simulink model "TLNWithUnrealTestBench"  (R2023a)
settings: Solver=FixedStepAuto  StartTime=0.0  StopTime=15  FixedStep=0.001  RelTol=1e-8  EnableMultiTasking=on
PostLoadFcn:
  | helperSLTrafficLightNegotiationWithUnrealSetup
values from neighbouring files (symbols this model uses):
  vehSim3D = repmat(     struct(     'Length', 0,     'InitialPos',[0 0 0],     'InitialRot',[0 0 0]),     numVehicles,1)    [helperSLTrafficLightNegotiationWithUnrealSetup.m]
undefined symbols (not defined in the file or in its folder): Curvature, CurvatureDerivative, driving, gray, HeadingAngle, intersectionInfo, LateralOffset, Left, M, matlabshared, N, referencePathInfo, Right, setVelocity, Strength, trafficLightConfig, Ts
libraries: drivingscenarioandsensors x8, sim3dautolib x4, visionanalysis x2, sim3dcameralib x2, sim3dlib x1, helperTrafficLightControllerLib x1, dspvision x1, trackingutilitieslib x1, drivinglib x1
CloseFcn:
  | helperSLTrafficLightNegotiationWithUnrealCleanUp
settings Model: Creator=The MathWorks, Inc.  LastModifiedBy=david
settings SolverCC: ZeroCrossAlgorithm=Adaptive  AlgebraicLoopSolver=TrustRegion  PositivePriorityOrder=on  AutoInsertRateTranBlk=on  InsertRTBMode=Always  DecoupledContinuousIntegration=on  MinimalZcImpactIntegration=on  MaxZcPerStep=1
settings DataIOCC: SaveOutput=off  SaveTime=off  ReturnWorkspaceOutputs=off
settings OptimizationCC: DefaultParameterBehavior=Inlined  EnhancedBackFolding=on  PassReuseOutputArgsAs=Individual arguments  ZeroExternalMemoryAtStartup=off  ZeroInternalMemoryAtStartup=off  OptimizeBlockOrder=speed  DifferentSizesBufferReuse=on  OptimizationCustomize=off  EfficientTunableParamExpr=on
settings DebuggingCC: MaskedZcDiagnostic=none  IgnoredZcDiagnostic=none  ParameterPrecisionLossMsg=none  ParameterTunabilityLossMsg=error  UnconnectedInputMsg=warning  UnconnectedOutputMsg=warning  UnconnectedLineMsg=warning  PregeneratedLibrarySubsystemCodeDiagnostic=none  ArithmeticOperatorsInVariantConditions=warning
settings HardwareCC: ProdLongLongMode=on
settings ModelReferenceCC: EnableRefExpFcnMdlSchedulingChecks=on
settings SFSimCC: SimUseLocalCustomCode=off
settings RTWCC: Description=Embedded Coder  SystemTargetFile=ert.tlc  TemplateMakefile=ert_default_tmf  GenerateReport=on  RTWUseLocalCustomCode=off  LaunchReport=on  DLArmComputeVersion=19.05
settings CodeAppCC: ForceParamTrailComments=on  IgnoreCustomStorageClasses=off  OperatorAnnotations=on  SimulinkDataObjDesc=on  SFDataObjDesc=on  InsertBlockDesc=on
settings ERTTargetCC: TargetLangStandard=C99 (ISO)  GenerateSampleERTMain=on  InlinedParameterPlacement=NonHierarchical  ERTCustomFileTemplate=example_file_process.tlc
settings ConfigComp: CovScope=ReferencedModels  CovIncludeTopModel=off

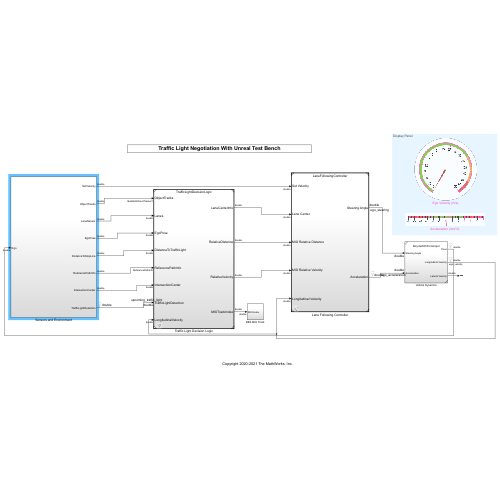
[thumbnail: Simulink's stored preview of the top-level diagram]
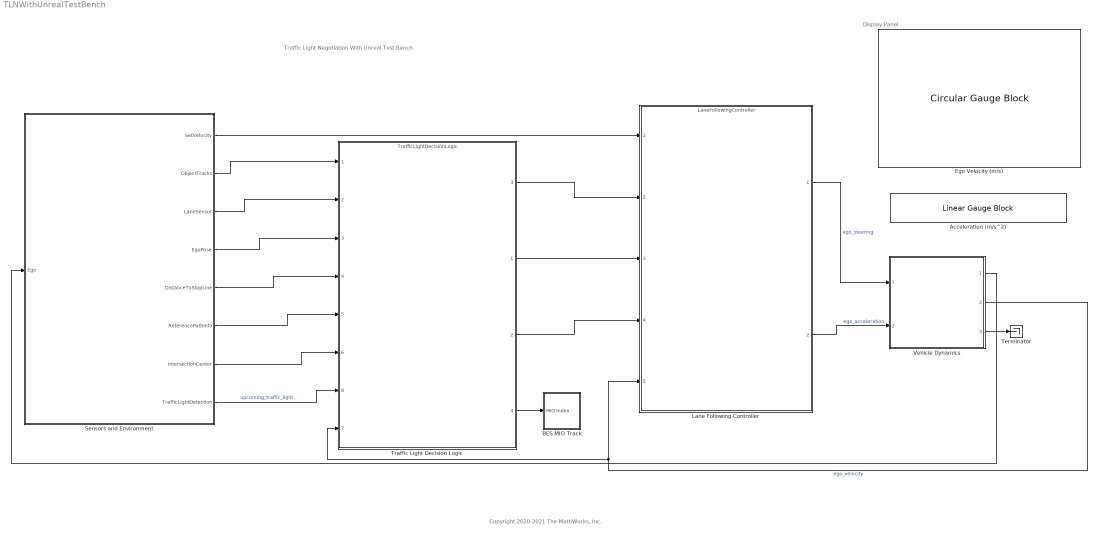
== system TLNWithUnrealTestBench ==
  note: Traffic Light Negotiation With Unreal Test Bench
  note: Display Panel
  note: Copyright 2020-2021 The MathWorks, Inc.
  Acceleration (m/s^2) : LinearGaugeBlock  LabelPosition=Hide  ScaleMin=-6  ScaleMax=6
  BES MIO Track : Subsystem
  Ego Velocity (m/s) : CircularGaugeBlock  LabelPosition=Hide  ScaleMax=50
  Lane Following Controller : ModelReference  ModelNameDialog=LaneFollowingController.slx  SimulationMode=Normal  ModelReferenceVersion=7.0
  Sensors and Environment : Subsystem
  Terminator : Terminator
  Traffic Light Decision Logic : ModelReference  ModelNameDialog=TrafficLightDecisionLogic  SimulationMode=Normal  ModelReferenceVersion=6.4
      settings: PortSchema="{\"entries\":[{\"content\":{\"sides\":[{\"content\":{\"connectorIds\":[\"In1\",\"In2\",\"In3\",\"In4\",\"In5\",\"In6\",\"In8\",\"In7\"]},\"type\":\"ConnectorPlacement.EquallySpacedRectSide\",\"uuid\":\"80441088-7f88-498e-bd57-56a9591db5ab\"},{\"content\":{\"connectorIds\":[\"Out3\",\"Out1\",\"Out2\",\"Out4\"],\"side\":\"RIGHT\"},\"type\":\"ConnectorPlacement.EquallySpacedRectSide\",\"uuid\":\"71bac071-b53b-4fb3-8fe7-17db6e81a6fe\"},{\"content\":{\"side\":\"TOP\"},\"type\":\"ConnectorPlacement.EquallySpacedRectSide\",\"uuid\":\"95fcddf4-1608-4cb5-a6ec-8633d9712dcc\"},{\"content\":{\"side\":\"HIDDEN\"},\"type\":\"ConnectorPlacement.EquallySpacedRectSide\",\"uuid\":\"8d5e9fdd-dbcd-4e58-97a7-7da238f3d39d\"}]},\"type\":\"ConnectorPlacement.EquallySpacedConnector\",\"uuid\":\"78ce1c2f-8a23-470e-877e-968badbfaf17\"}],\"packageUris\":[\"http://schema.mathworks.com/mf0/Connector/R2020b\"],\"version\":\"1.0\"}"
  Vehicle Dynamics : Subsystem  ReferencedSubsystem=BicycleWithForceInput
  wires:
  Sensors and Environment/2(ObjectTracks) -> Traffic Light Decision Logic/1
  Sensors and Environment/1(SetVelocity) -> Lane Following Controller/1
  Sensors and Environment/8(TrafficLightDetection) -> Traffic Light Decision Logic/8  "upcoming_traffic_light"
  Vehicle Dynamics/1 -> Sensors and Environment/1(Ego)
  Sensors and Environment/4(EgoPose) -> Traffic Light Decision Logic/3
  Sensors and Environment/3(LaneSensor) -> Traffic Light Decision Logic/2
  Sensors and Environment/5(DistanceToStopLine) -> Traffic Light Decision Logic/4
  Sensors and Environment/6(ReferencePathInfo) -> Traffic Light Decision Logic/5
  Sensors and Environment/7(IntersectionCenter) -> Traffic Light Decision Logic/6
  Lane Following Controller/1 -> Vehicle Dynamics/1  "ego_steering"
  Lane Following Controller/2 -> Vehicle Dynamics/2  "ego_acceleration"
  Traffic Light Decision Logic/3 -> Lane Following Controller/2
  Traffic Light Decision Logic/1 -> Lane Following Controller/3
  Traffic Light Decision Logic/2 -> Lane Following Controller/4
  Traffic Light Decision Logic/4 -> BES MIO Track/1(MIO Index)
  Vehicle Dynamics/2 -> Lane Following Controller/5, Traffic Light Decision Logic/7  "ego_velocity"
  Vehicle Dynamics/3 -> Terminator/1

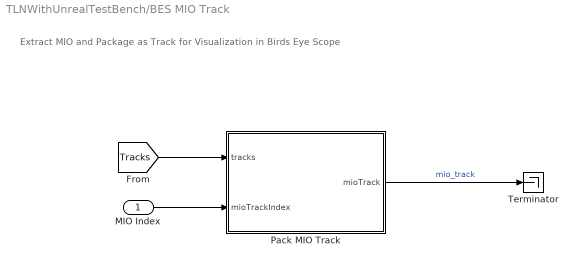
== system TLNWithUnrealTestBench/BES MIO Track ==
  note: Extract MIO and Package as Track for Visualization in Birds Eye Scope
  MIO Index : Inport
  Pack MIO Track : MATLAB Function  TreatAsAtomicUnit=on
  Terminator : Terminator
  wires:
  MIO Index/1 -> Pack MIO Track/2(mioTrackIndex)
  [Tracks] -> Pack MIO Track/1(tracks)
  Pack MIO Track/1(mioTrack) -> Terminator/1  "mio_track"

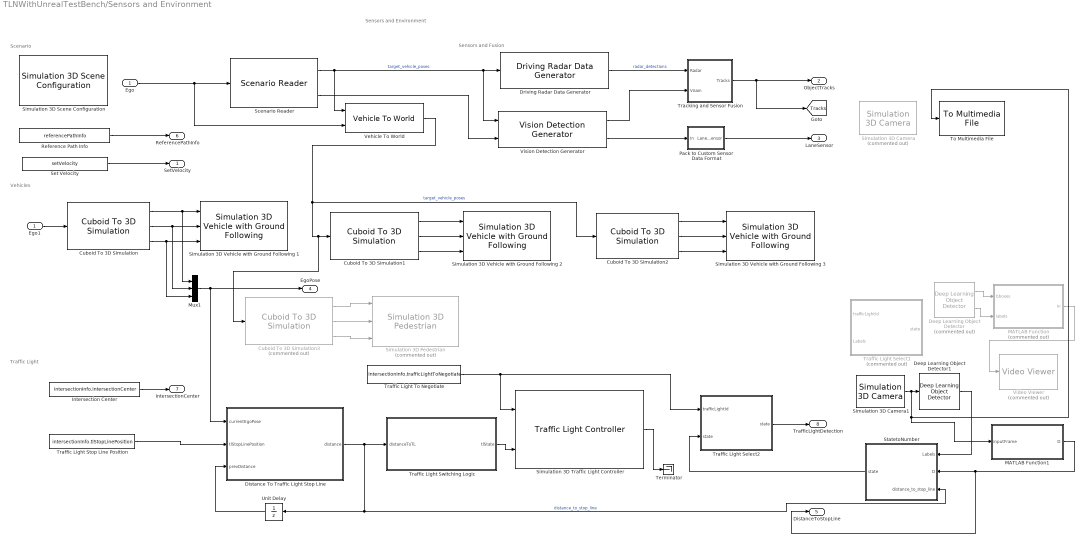
== system TLNWithUnrealTestBench/Sensors and Environment ==
  note: Sensors and Fusion
  note: Traffic Light
  note: Scenario
  note: Sensors and Environment
  note: Vehicles
  Ego : Inport
  Cuboid To 3D Simulation : drivingscenarioandsensors/Cuboid To 3D Simulation  SpecifyActorID=off  ActorIDToConvert=1  SimulateUsing=Interpreted execution
  Cuboid To 3D Simulation1 : drivingscenarioandsensors/Cuboid To 3D Simulation  SpecifyActorID=on  ActorIDToConvert=68  SimulateUsing=Interpreted execution
  Cuboid To 3D Simulation2 : drivingscenarioandsensors/Cuboid To 3D Simulation  SpecifyActorID=on  ActorIDToConvert=69  SimulateUsing=Interpreted execution
  Cuboid To 3D Simulation3 : drivingscenarioandsensors/Cuboid To 3D Simulation  Commented=on  SpecifyActorID=on  ActorIDToConvert=70  SimulateUsing=Interpreted execution
  Deep Learning Object Detector : visionanalysis/Deep Learning Object Detector  Commented=on  Detector=Detector from MAT-file  DetectorFunction=untitled  DetectorFilePath=C:\Users\david\Documents\MATLAB\TLNUnreal\TLNUnreal\TestAnalysis\Training_GYR\DetectorYolov2.mat  MaxDetections=500  Bboxes=on  Scores=off  UseROI=off  ROI=[1 1 100 100]  Threshold=0.5  NumStrongestRegions=2000  UseMinSize=off  MinSize=[1 1]  UseMaxSize=off  MaxSize=[50 50]  ForceInterpretedSim=off
  Deep Learning Object Detector1 : visionanalysis/Deep Learning Object Detector  Detector=Detector from MAT-file  DetectorFunction=untitled  DetectorFilePath=C:\Users\david\Documents\MATLAB\TLNUnreal\TLNUnreal\NoState\detectorYolo2.mat  MaxDetections=500  Bboxes=off  Scores=off  UseROI=off  ROI=[1 1 100 100]  Threshold=0.5  NumStrongestRegions=2000  UseMinSize=off  MinSize=[1 1]  UseMaxSize=off  MaxSize=[50 50]  ForceInterpretedSim=off
  Distance To Traffic Light Stop Line : MATLAB Function  TreatAsAtomicUnit=on  mask{minTLDist=3}
      mask prompts: minTLDist "Minimum distance to traffic light"
  Driving Radar Data Generator : drivingscenarioandsensors/Driving Radar Data Generator  SensorIndex=2  UpdateRate=10  MountingLocation=[ 0, 0.5, 0.2 ]  MountingAngles=[0 0 0]  HasElevation=off  HasRangeRate=on  HasNoise=off  HasFalseAlarms=off  HasOcclusion=on  MaxNumReportsSource=Property  MaxNumReports=50  TargetReportFormat=Clustered detections  DetectionCoordinates=Body  TrackCoordinates=Body  BusNameSource=Property  BusName=BusRadar  AzimuthResolution=4  ElevationResolution=5  RangeResolution=2.5  RangeRateResolution=0.5  AzimuthBiasFraction=0.1  ElevationBiasFraction=0.1  RangeBiasFraction=0.05  RangeRateBiasFraction=0.05  FieldOfView=[40, 5 ]  RangeLimits=[ 0, 174 ]  RangeRateLimits=[ -100, 100 ]  DetectionProbability=0.9  FalseAlarmRate=1e-06  ReferenceRange=100  ReferenceRCS=0  CenterFrequency=77e9  FilterInitializationFcn=initcvekf  ConfirmationThreshold=[2 3]  DeletionThreshold=[5 5]  InitialSeedSource=Repeatable  InitialSeed=0  UsedSeed=matlabshared.tracking.internal.SimulinkUtilities.seedManager(gcb)  ProfilesSource=From Scenario Reader block  ProfilesParameters=driving.internal.ActorProfilesRadarParameters  ProfilesExpression=struct('ClassID',0,'Length',4.7,'Width',1.8,'Height',1.4,'OriginOffset',[-1.35 0 0],'RCSPattern',[10 10;10 10],'RCSAzimuthAngles',[-180 180],'RCSElevationAngles',[-90 90])
  Ego1 : InportShadow
  Intersection Center : Constant  Value=intersectionInfo.intersectionCenter  SampleTime=Ts
  MATLAB Function : MATLAB Function  Commented=on  TreatAsAtomicUnit=on
  MATLAB Function1 : MATLAB Function  TreatAsAtomicUnit=on
  Mux1 : Mux  Inputs=3
  Pack to Custom Sensor Data Format : Subsystem
  Reference Path Info : Constant  Value=referencePathInfo  OutDataTypeStr=Bus: ReferencePathInfo  SampleTime=Ts
  Scenario Reader : drivingscenarioandsensors/Scenario Reader  ScenarioSource=From workspace  ScenarioFileName=C:\Users\david\Documents\MATLAB\TLNUnreal\TLNUnreal\TestScenarios\90DegreesStraight.mat  ScenarioVariableName=scenario_02_TLN_straight_greenToRed  OutputCoordinateSystem=Vehicle coordinates  EgoVehicleSource=Input port  EgoVehicleActorID=egoVehicle.ActorID  OrientVehiclesOnRoad=on  OutputEgoVehiclePose=off  OutputEgoVehicleState=off  SampleTime=Ts  LaneBoundaryOutput=All lane boundaries  LaneBoundaryDistance=0:0.5:60  LaneBoundaryLocation=Center of lane markings  BusNameSource=Auto  BusName=BusActors  BusNumActorsSource=Scenario  BusNumActors=100  BusName2Source=Auto  BusName2=BusLaneBoundaries  BusNumLaneBoundariesSource=Scenario  BusNumLaneBoundaries=10  BusName3Source=Auto  BusName3=BusEgoActor  BusName4Source=Auto  BusName4=BusEgoState  ShowCoordinateLabels=on  SimulateUsing=Interpreted execution
  Set Velocity : Constant  Value=setVelocity
  Simulation 3D Camera : sim3dcameralib/Simulation 3D Camera  Priority=1  Commented=on  sensorTag=Sim3dSensor3  sensorId=3  sensorName=Sim3dSensor3  vehTagList={'EgoVehicle';'Scene Origin';'SimulinkVehicle2';'SimulinkVehicle3'}  vehTag=EgoVehicle  mountLoc=Roof center  offsetFlag=off  tmountOffset=[0, 0, 0]  extTmount=off  rmountOffset=[0, 0, 0]  extRmount=off  FocalLength=[1109, 1109]  OpticalCenter=[640, 360]  ImageSize=[720, 1280]  RadialDistortion=[0, 0]  TangentialDistortion=[0, 0]  SensorSkew=0  DepthOutportEnabled=off  SemanticOutportEnabled=off  TransformOutportEnabled=off  SampleTime=-1  mountPoint=[-0.449999988079071 0 1.67999994754791]  mountOrientation=[0 0 0]  aMode=3  ID=3
      settings: LibrarySourceBlock=drivingsim3d/Simulation 3D Camera
  Simulation 3D Camera1 : sim3dcameralib/Simulation 3D Camera  Priority=1  sensorTag=Sim3dSensor2  sensorId=2  sensorName=Sim3dSensor2  vehTagList={'EgoVehicle';'Scene Origin';'SimulinkVehicle2';'SimulinkVehicle3'}  vehTag=EgoVehicle  mountLoc=Roof center  offsetFlag=off  tmountOffset=[0, 0, 0]  extTmount=off  rmountOffset=[0, 0, 0]  extRmount=off  FocalLength=[1109, 1109]  OpticalCenter=[640, 360]  ImageSize=[720, 1280]  RadialDistortion=[0, 0]  TangentialDistortion=[0, 0]  SensorSkew=0  DepthOutportEnabled=off  SemanticOutportEnabled=off  TransformOutportEnabled=off  SampleTime=-1  mountPoint=[-0.449999988079071 0 1.67999994754791]  mountOrientation=[0 0 0]  aMode=3  ID=2
      settings: LibrarySourceBlock=drivingsim3d/Simulation 3D Camera
  Simulation 3D Pedestrian : sim3dautolib/Simulation 3D Pedestrian  Priority=-1  Commented=on  PedestrianType=Male 1  Scale=[1, 1, 1]  InitialPos=[-55.1, -4, 0]  InitialYaw=0  ActorName=SimulinkPedestrian1  SampleTime=-1  ActorType=SimulinkPedestrian  ActorTag=SimulinkPedestrian1  ID=1  aMode=3  CoordinateScheme=ISO  TransformOutportEnabled=off
      settings: LibrarySourceBlock=drivingsim3d/Simulation 3D Pedestrian
  Simulation 3D Scene Configuration : sim3dlib/Simulation 3D Scene Configuration  Priority=0  ProjectFormat=Unreal Executable  SceneDesc=US city block  ProjectName=C:\Users\david\Documents\MATLAB\NoLightOn\WindowsNoEditor\AutoVrtlEnv.exe  ScenePath=/Game/Maps/USCityBlock  UEProjPath=C:\Users\david\Documents\MATLAB\AutoVrtlEnv - Copy\AutoVrtlEnv.uproject  EnableOpenDRIVE=off  vehTagList={'EgoVehicle';'Scene Origin';'SimulinkVehicle2';'SimulinkVehicle3'}  vehTag=EgoVehicle  OpVisEn=off  Ts=0.1  EnableWindow=on  EnableRemoteAccess=off  EnableWeather=off  SunAltitude=40.0  SunAzimuth=90  clouds=10  wind=1  fog=0  rain=0  EnableGeospatial=off  OriginHeight=200  OriginLatitude=40.744652  OriginLongitude=-73.988864  MapStyle=Aerial  AdditionalAssetIDs=[]  UseAdvancedSunSky=off  SolarTime=11  TimeZone=-5  Day=21  Month=9  Year=2022  UseDaylightSavingTime=on  DSTStartDay=10  DSTStartMonth=3  DSTEndDay=3  DSTEndMonth=11  DSTSwitchHour=2  sensorTag=MainCamera1  sensorId=1  sensorName=MainCamera1  mountLoc=Origin  offsetFlag=off  tmountOffset=[0, 0, 0]  rmountOffset=[0, 0, 0]  HorizontalResolution=1280  VerticalResolution=720  HorizontalFOV=60  mountPoint=[0 0 0]  mountOrientation=[0 0 0]  aMode=3  ID=1  GeoTrigger=Inactive
      settings: AttributesFormatString=SceneDesc = %<SceneDesc>
  Simulation 3D Traffic Light Controller : helperTrafficLightControllerLib/Traffic Light Controller  Priority=-1  helperTrafficLightCheck=0  customScene=0  modeType=State-based  vehTagList={'EgoVehicle';'Scene Origin';'SimulinkVehicle2';'SimulinkVehicle3'}  MsgSize=[1 62]  vehTag=EgoVehicle  trafficLightID=1  greenTime=10  yellowTime=3  redClearanceTime=0  aMode=3  Ts=-1
  Simulation 3D Vehicle with Ground Following 1 : sim3dautolib/Simulation 3D Vehicle with Ground Following  Priority=-1  PassVehMesh=Sedan  MeshPath=/MathWorksSimulation/Vehicles/Muscle/Meshes/SK_MuscleCar.SK_MuscleCar  TrackWidth=1.9  WheelBase=3  WheelRadius=0.35  VehColor=Blue  InitialPos=vehSim3D(1).InitialPos  InitialRot=vehSim3D(1).InitialRot  ActorName=EgoVehicle  SampleTime=-1  ActorType=SimulinkVehicle  ID=C  aMode=3  ActorTag=EgoVehicle  CoordinateScheme=ISO  VehLightsControl=off  HeadlightColor=[ 1, 1, 1 ]  HighBeamIntensity=100000  LowBeamIntensity=60000  HighBeamConeAngle=70  LowBeamConeAngle=70  LeftHeadlightOrientation=[ 0, 0 ]  RightHeadlightOrientation=[ 0, 0 ]  BrakelightIntensity=500  ReverselightIntensity=500  SignallightIntensity=500  SignallightPeriod=1  SignalPulseWidth=50  TransformOutportEnabled=off
      settings: AttributesFormatString=|
      | --------------------------------------
      | ActorName = %<ActorName>
      | PassVehMesh = %<PassVehMesh>
      | VehColor = %<VehColor>
  Simulation 3D Vehicle with Ground Following 2 : sim3dautolib/Simulation 3D Vehicle with Ground Following  Priority=-1  PassVehMesh=Sedan  MeshPath=/MathWorksSimulation/Vehicles/Muscle/Meshes/SK_MuscleCar.SK_MuscleCar  TrackWidth=1.9  WheelBase=3  WheelRadius=0.35  VehColor=Red  InitialPos=vehSim3D(2).InitialPos  InitialRot=vehSim3D(2).InitialRot  ActorName=SimulinkVehicle2  SampleTime=-1  ActorType=SimulinkVehicle  ID=2  aMode=3  ActorTag=SimulinkVehicle2  CoordinateScheme=ISO  VehLightsControl=off  HeadlightColor=[ 1, 1, 1 ]  HighBeamIntensity=100000  LowBeamIntensity=60000  HighBeamConeAngle=70  LowBeamConeAngle=70  LeftHeadlightOrientation=[ 0, 0 ]  RightHeadlightOrientation=[ 0, 0 ]  BrakelightIntensity=500  ReverselightIntensity=500  SignallightIntensity=500  SignallightPeriod=1  SignalPulseWidth=50  TransformOutportEnabled=off
      settings: AttributesFormatString=|
      | --------------------------------------
      | ActorName = %<ActorName>
      | PassVehMesh = %<PassVehMesh>
      | VehColor = %<VehColor>
  Simulation 3D Vehicle with Ground Following 3 : sim3dautolib/Simulation 3D Vehicle with Ground Following  Priority=-1  PassVehMesh=Muscle car  MeshPath=/MathWorksSimulation/Vehicles/Muscle/Meshes/SK_MuscleCar.SK_MuscleCar  TrackWidth=1.9  WheelBase=3  WheelRadius=0.35  VehColor=Black  InitialPos=vehSim3D(3).InitialPos  InitialRot=vehSim3D(3).InitialRot  ActorName=SimulinkVehicle3  SampleTime=-1  ActorType=SimulinkVehicle  ID=3  aMode=3  ActorTag=SimulinkVehicle3  CoordinateScheme=ISO  VehLightsControl=off  HeadlightColor=[ 1, 1, 1 ]  HighBeamIntensity=100000  LowBeamIntensity=60000  HighBeamConeAngle=70  LowBeamConeAngle=70  LeftHeadlightOrientation=[ 0, 0 ]  RightHeadlightOrientation=[ 0, 0 ]  BrakelightIntensity=500  ReverselightIntensity=500  SignallightIntensity=500  SignallightPeriod=1  SignalPulseWidth=50  TransformOutportEnabled=off
      settings: AttributesFormatString=|
      | --------------------------------------
      | ActorName = %<ActorName>
      | PassVehMesh = %<PassVehMesh>
      | VehColor = %<VehColor>
  StatetoNumber : MATLAB Function  TreatAsAtomicUnit=on
  Terminator : Terminator
  To Multimedia File : dspvision/To Multimedia File  outputFilename=C:\Users\david\Documents\MATLAB\Presentation\Gree,Yellow,Red.avi  streamSelection=Video only  videoCompressor=None (uncompressed)  audioCompressor=None (uncompressed)  imagePorts=One multidimensional signal  fileType=AVI  audioDatatype=Determine from input data type  fourcc=RGB  videoQuality=75  mj2000CompFactor=10
      settings: LibrarySourceBlock=visionsinks/To Multimedia File
  Tracking and Sensor Fusion : Subsystem  TreatAsAtomicUnit=on
      settings: RTWFileNameOpts=Use function name
  Traffic Light Select1 : MATLAB Function  Commented=on  TreatAsAtomicUnit=on
  Traffic Light Select2 : MATLAB Function  TreatAsAtomicUnit=on
  Traffic Light Stop Line Position : Constant  Value=intersectionInfo.tlStopLinePosition  OutDataTypeStr=double
  Traffic Light Switching Logic : Stateflow chart  TreatAsAtomicUnit=on  SystemSampleTime=Ts  mask{tlConfig=trafficLightConfig}
      mask prompts: tlConfig "Configuration Params"
  Traffic Light To Negotiate : Constant  Value=intersectionInfo.trafficLightToNegotiate
  Unit Delay : UnitDelay  InitialCondition=100  SampleTime=-1  HasFrameUpgradeWarning=on
  Vehicle To World : drivingscenarioandsensors/Vehicle To World  BusNameSource=Auto  BusName=BusVehicleToWorldActors  SimulateUsing=Interpreted execution
  Video Viewer : VideoViewer  Commented=on  colormapValue=gray(256)  FigPos=[1 726 1366 626]
  Vision Detection Generator : drivingscenarioandsensors/Vision Detection Generator  SensorIndex=1  DetectorOutput=Lanes and objects  UpdateInterval=0.1  LaneUpdateInterval=0.1  SensorLocation=[ 1.9, 0 ]  Height=1.1  Yaw=0  Pitch=1  Roll=0  BusNameSource=Property  BusName=BusVision  BusName2Source=Property  BusName2=BusLanes  MaxNumDetectionsSource=Property  MaxNumDetections=20  MaxNumLanesSource=Property  MaxNumLanes=2  DetectionCoordinates=Ego Cartesian  SimulateUsing=Interpreted execution  MaxRange=150  BoundingBoxAccuracy=5  ProcessNoiseIntensity=5  MaxSpeed=50  MaxAllowedOcclusion=0.5  MinObjectImageSize=[ 10, 10 ]  DetectionProbability=0.9  FalsePositivesPerImage=0.1  MinLaneImageSize=[ 20, 3 ]  LaneBoundaryAccuracy=3  HasNoise=on  InitialSeedSource=Repeatable  InitialSeed=0  UsedSeed=driving.internal.SimulinkUtilities.seedManager(gcb)  ActorProfilesSource=From Scenario Reader block  ActorProfilesParameters=driving.internal.ActorProfilesParameters  ActorProfilesExpression=struct( 'ClassID', 0, 'Length', 4.7, 'Width', 1.8, 'Height', 1.4, 'OriginOffset', [ -1.35, 0, 0 ] )  Intrinsics=driving.internal.cameraIntrinsics('FocalLength',[ 800,800 ])
  SetVelocity : Outport
  ObjectTracks : Outport  Port=2
  LaneSensor : Outport  Port=3  VectorParamsAs1DForOutWhenUnconnected=off
  EgoPose : Outport  Port=4
  DistanceToStopLine : Outport  Port=5
  ReferencePathInfo : Outport  Port=6
  IntersectionCenter : Outport  Port=7
  TrafficLightDetection : Outport  Port=8  SampleTime=Ts
  tag scope: Tracks=global
  wires:
  Scenario Reader/1 -> Vehicle To World/1, Driving Radar Data Generator/1, Vision Detection Generator/1  "target_vehicle_poses"
  Cuboid To 3D Simulation1/3 -> Simulation 3D Vehicle with Ground Following 2/3
  Cuboid To 3D Simulation1/2 -> Simulation 3D Vehicle with Ground Following 2/2
  Cuboid To 3D Simulation2/2 -> Simulation 3D Vehicle with Ground Following 3/2
  Cuboid To 3D Simulation2/3 -> Simulation 3D Vehicle with Ground Following 3/3
  Vehicle To World/1 -> Cuboid To 3D Simulation3/1, Cuboid To 3D Simulation1/1, Cuboid To 3D Simulation2/1  "target_vehicle_poses"
  Cuboid To 3D Simulation1/1 -> Simulation 3D Vehicle with Ground Following 2/1
  Cuboid To 3D Simulation2/1 -> Simulation 3D Vehicle with Ground Following 3/1
  Scenario Reader/2 -> Vision Detection Generator/2
  Tracking and Sensor Fusion/1(Tracks) -> [Tracks], ObjectTracks/1
  Vision Detection Generator/2 -> Pack to Custom Sensor Data Format/1(In)
  Pack to Custom Sensor Data Format/1(LaneSensor) -> LaneSensor/1
  Traffic Light Stop Line Position/1 -> Distance To Traffic Light Stop Line/2(tlStopLinePosition)
  Traffic Light Select2/1(state) -> TrafficLightDetection/1
  Ego/1 -> Scenario Reader/1, Vehicle To World/2
  Ego1/1 -> Cuboid To 3D Simulation/1
  Cuboid To 3D Simulation/2 -> Mux1/2, Simulation 3D Vehicle with Ground Following 1/2
  Cuboid To 3D Simulation/1 -> Mux1/1, Simulation 3D Vehicle with Ground Following 1/1
  Cuboid To 3D Simulation/3 -> Mux1/3, Simulation 3D Vehicle with Ground Following 1/3
  Distance To Traffic Light Stop Line/1(distance) -> Traffic Light Switching Logic/1(distanceToTL), StatetoNumber/3(distance_to_stop_line), Unit Delay/1  "distance_to_stop_line"
  Mux1/1 -> EgoPose/1, Distance To Traffic Light Stop Line/1(currentEgoPose)
  Traffic Light To Negotiate/1 -> Simulation 3D Traffic Light Controller/1, Traffic Light Select2/1(trafficLightId)
  Intersection Center/1 -> IntersectionCenter/1
  Unit Delay/1 -> Distance To Traffic Light Stop Line/3(prevDistance)
  Reference Path Info/1 -> ReferencePathInfo/1
  Set Velocity/1 -> SetVelocity/1
  Deep Learning Object Detector/1 -> MATLAB Function/1(bboxes)
  Deep Learning Object Detector/2 -> MATLAB Function/2(labels)
  MATLAB Function/1(In) -> Video Viewer/1
  Deep Learning Object Detector1/1 -> StatetoNumber/1(Labels)
  Simulation 3D Traffic Light Controller/1 -> Terminator/1
  Traffic Light Switching Logic/1(tlState) -> Simulation 3D Traffic Light Controller/2
  StatetoNumber/1(state) -> Traffic Light Select2/2("state ")
  Cuboid To 3D Simulation3/1 -> Simulation 3D Pedestrian/1
  Cuboid To 3D Simulation3/2 -> Simulation 3D Pedestrian/2
  Cuboid To 3D Simulation3/3 -> Simulation 3D Pedestrian/3
  Vision Detection Generator/1 -> Tracking and Sensor Fusion/2(Vision)
  Driving Radar Data Generator/1 -> Tracking and Sensor Fusion/1(Radar)  "radar_detections"
  Simulation 3D Camera1/1 -> To Multimedia File/1, MATLAB Function1/1(inputFrame), Deep Learning Object Detector1/1
  ? -> ?
  MATLAB Function1/1(D) -> DistanceToStopLine/1, StatetoNumber/2(D)

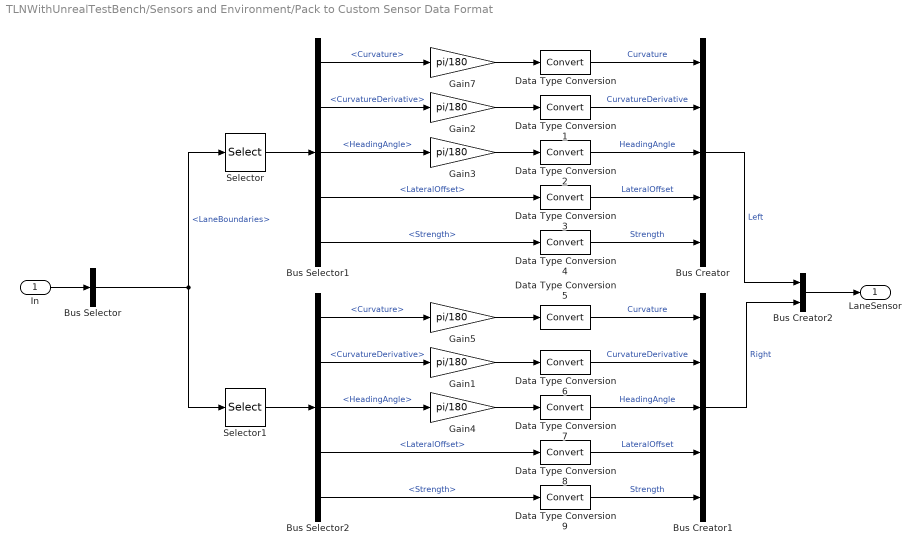
== system TLNWithUnrealTestBench/Sensors and Environment/Pack to Custom Sensor Data Format ==
  In : Inport
  Bus Creator : BusCreator  Inputs=Curvature,CurvatureDerivative,HeadingAngle,LateralOffset,Strength  OutDataTypeStr=Bus: LaneSensorBoundaries
  Bus Creator1 : BusCreator  Inputs=Curvature,CurvatureDerivative,HeadingAngle,LateralOffset,Strength  OutDataTypeStr=Bus: LaneSensorBoundaries
  Bus Creator2 : BusCreator  Inputs=Left,Right  OutDataTypeStr=Bus: LaneSensor
  Bus Selector : BusSelector  OutputSignals=LaneBoundaries
  Bus Selector1 : BusSelector  OutputSignals=Curvature,CurvatureDerivative,HeadingAngle,LateralOffset,Strength
  Bus Selector2 : BusSelector  OutputSignals=Curvature,CurvatureDerivative,HeadingAngle,LateralOffset,Strength
  Data Type Conversion{,1..9} (10 alike) : DataTypeConversion  SaturateOnIntegerOverflow=off  RndMeth=Floor
  Gain{1..5,7} (6 alike) : Gain  Gain=pi/180
  Selector : Selector  InputPortWidth=2  IndexOptions=Index vector (dialog)  Indices=1  OutputSizes=1
  Selector1 : Selector  InputPortWidth=2  IndexOptions=Index vector (dialog)  Indices=2  OutputSizes=1
  LaneSensor : Outport  VectorParamsAs1DForOutWhenUnconnected=off
  wires:
  In/1 -> Bus Selector/1
  Bus Selector/1 -> Selector/1, Selector1/1  "<LaneBoundaries>"
  Selector/1 -> Bus Selector1/1
  Bus Selector1/2 -> Gain2/1  "<CurvatureDerivative>"
  Bus Selector1/1 -> Gain7/1  "<Curvature>"
  Bus Selector1/3 -> Gain3/1  "<HeadingAngle>"
  Gain7/1 -> Data Type Conversion/1
  Gain2/1 -> Data Type Conversion1/1
  Gain3/1 -> Data Type Conversion2/1
  Bus Selector1/4 -> Data Type Conversion3/1  "<LateralOffset>"
  Bus Selector1/5 -> Data Type Conversion4/1  "<Strength>"
  Data Type Conversion/1 -> Bus Creator/1  "Curvature"
  Data Type Conversion1/1 -> Bus Creator/2  "CurvatureDerivative"
  Data Type Conversion2/1 -> Bus Creator/3  "HeadingAngle"
  Data Type Conversion3/1 -> Bus Creator/4  "LateralOffset"
  Data Type Conversion4/1 -> Bus Creator/5  "Strength"
  Data Type Conversion9/1 -> Bus Creator1/5  "Strength"
  Data Type Conversion6/1 -> Bus Creator1/2  "CurvatureDerivative"
  Data Type Conversion7/1 -> Bus Creator1/3  "HeadingAngle"
  Data Type Conversion8/1 -> Bus Creator1/4  "LateralOffset"
  Data Type Conversion5/1 -> Bus Creator1/1  "Curvature"
  Bus Selector2/1 -> Gain5/1  "<Curvature>"
  Selector1/1 -> Bus Selector2/1
  Bus Selector2/4 -> Data Type Conversion8/1  "<LateralOffset>"
  Bus Selector2/5 -> Data Type Conversion9/1  "<Strength>"
  Bus Selector2/2 -> Gain1/1  "<CurvatureDerivative>"
  Gain4/1 -> Data Type Conversion7/1
  Gain5/1 -> Data Type Conversion5/1
  Gain1/1 -> Data Type Conversion6/1
  Bus Selector2/3 -> Gain4/1  "<HeadingAngle>"
  Bus Creator2/1 -> LaneSensor/1
  Bus Creator/1 -> Bus Creator2/1  "Left"
  Bus Creator1/1 -> Bus Creator2/2  "Right"

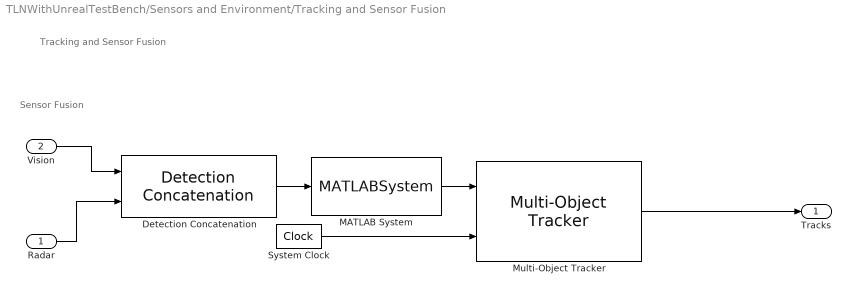
== system TLNWithUnrealTestBench/Sensors and Environment/Tracking and Sensor Fusion ==
  note: Tracking and Sensor Fusion
  note: Sensor Fusion
  Radar : Inport  OutDataTypeStr=Bus: BusRadar  PortDimensions=[1 1]  BusOutputAsStruct=on
  Vision : Inport  Port=2  OutDataTypeStr=Bus: BusVision  PortDimensions=[1 1]  BusOutputAsStruct=on
  Detection Concatenation : trackingutilitieslib/Detection Concatenation  NumInputs=2  BusNameSource=Auto  BusName=BusDetectionConcatenation  SimulateUsing=Interpreted execution
  MATLAB System : MATLABSystem  System=helperVehicleSize  VehicleSize=vehicleLength  BusNameSource=Auto  BusName=BusVehicleSizeDetections  SimulateUsing=Interpreted execution
      mask Type: helperVehicleSize
      mask Display:
      | disp('helperVehicleSize');
      | port_label('input',1,'In');
      | port_label('output',1,'Out');
  Multi-Object Tracker : drivinglib/Multi-Object Tracker  TrackerIndex=uint32( 0 )  FilterInitializationFcn=initcvekf  AssignmentThreshold=assigThresh  ConfirmationThreshold=[ M, N ]  DeletionThreshold=[ 5, 5 ]  MaxNumTracks=numTracks  MaxNumSensors=numSensors  OOSMHandling=Terminate  StateParametersSimulink=struct  HasStateParametersInput=off  TimeInputSource=Input port  HasCostMatrixInput=off  HasDetectableTrackIDsInput=off  BusNameSource=Property  BusName=BusMultiObjectTracker1  TentativeTracksOutputPort=off  AllTracksOutputPort=off  SimulateUsing=Interpreted execution
  System Clock : DigitalClock  SampleTime=Ts
  Tracks : Outport  OutDataTypeStr=Bus:BusMultiObjectTracker1  PortDimensions=[1 1]  VectorParamsAs1DForOutWhenUnconnected=off  BusOutputAsStruct=on
  wires:
  Detection Concatenation/1 -> MATLAB System/1
  Multi-Object Tracker/1 -> Tracks/1
  Radar/1 -> Detection Concatenation/2
  System Clock/1 -> Multi-Object Tracker/2
  Vision/1 -> Detection Concatenation/1
  MATLAB System/1 -> Multi-Object Tracker/1

== matlab function TLNWithUnrealTestBench/BES MIO Track/Pack MIO Track ==
  data: tracks input; mioTrack output Bus: BusMultiObjectTracker1; mioTrackIndex input
function mioTrack = fcn(tracks, mioTrackIndex)
% Extract MIO track and package for visualization in Birds Eye Scope

mioTrack = tracks;

if mioTrackIndex > 0
    % First track represents MIO
    mioTrack.NumTracks = 1;
    mioTrack.Tracks(1) = tracks.Tracks(mioTrackIndex);
else
    % No valid MIO track
    mioTrack.NumTracks = 0;
end

== matlab function TLNWithUnrealTestBench/Sensors and Environment/MATLAB Function ==
  data: bboxes input; labels input; In output
function In = lane_vehicle_annotation(bboxes,labels)

% Copyright 2020-2021 The MathWorks, Inc.

if ~isempty(labels)
    In = labels;
end

% function In = lane_vehicle_annotation(bboxes,labels,In)
% 
% % Copyright 2020-2021 The MathWorks, Inc.
% 
% if ~isempty(bboxes)
%     In = insertObjectAnnotation(In, 'rectangle',bboxes,labels);
% end

== matlab function TLNWithUnrealTestBench/Sensors and Environment/MATLAB Function1 ==
  data: inputFrame input; D output
function D = processCameraFrame(inputFrame)
img = inputFrame; 
grayImg = rgb2gray(img);

% Get the size of the original image
[height, width, ~] = size(img);

% Define the ROI for the left half up to the center
roi_x = 1 :width;
roi_y = (3*height/5):height-20;

% Crop the image to the defined ROI
croppedImg = img(roi_y, roi_x, :);

% Load the image
img = croppedImg;

% Convert the image to grayscale (if not already)
grayImg = rgb2gray(img);

%Smoothing the image
img_smoothed = imgaussfilt(grayImg, 2.5); % Adjust the standard deviation as needed
img_enhanced = histeq(img_smoothed);%Enhance technique

%Edge detection
img_edges = edge(img_enhanced, 'Canny');
se = strel('line', 3, 45); % Adjust the structuring element based on the requirements
img_edges_dilated = imdilate(img_edges, se);
edgeImg = img_edges_dilated; 

% Perform the Hough Transform
[H, theta, rho] = hough(edgeImg);

% Find peaks in the Hough Transform
numPeaks = 10;  % You can adjust the number of peaks to detect
peaks = houghpeaks(H, numPeaks);

% Extract lines based on the peaks
lines = houghlines(edgeImg, theta, rho, peaks);

% Load the image and perform line detection as previously described

% Define the angle range for the specific line you want to detect
angleRange = [-90, -80]; % Adjust this range as needed

% Define the minimum and maximum line length (in pixels)
minLineLength = 421; % Adjust as needed
maxLineLength = 980; % Adjust as needed


% Initialize an empty array to store the specific lines
specificLines = [];

% Iterate through the detected lines and filter based on angle and length
for i = 1:length(lines)
    angle = lines(i).theta; % Get the angle of the line
    lineLength = norm(lines(i).point1 - lines(i).point2); % Calculate line length
    
    % Check if the angle falls within the specified range and line length is within the specified range
    if angle >= angleRange(1) && angle <= angleRange(2) && ...
       lineLength >= minLineLength && lineLength <= maxLineLength;
        specificLines = [specificLines, lines(i)];
    end
end

% Assuming you want to calculate the distance for a specific line (e.g., the first line in specificLines)
% Make sure that specificLines is not empty

if ~isempty(specificLines)
    % Extract the specific line you are interested in
    specificLine = specificLines(1); % Change the index if needed

    % Extract endpoints of the specific line
    x1 = specificLine.point1(1);
    y1 = specificLine.point1(2);
    x2 = specificLine.point2(1);
    y2 = specificLine.point2(2);

    % Calculate PixelLineLength
    PixelLineLength = sqrt((x2 - x1)^2 + (y2 - y1)^2);

    % Given parameters
    FocalLength = 1190; %same for x and y
    SensorHeight = 360;
    width = 6;

    % Calculate the distance (D)

    D = FocalLength*width / PixelLineLength;
    % Display the distance
else
    D = Inf;
end

== matlab function TLNWithUnrealTestBench/Sensors and Environment/Distance To Traffic Light Stop Line ==
  data: currentEgoPose input; tlStopLinePosition input; prevDistance input; distance output; minTLDist parameter
function distance   = distanceToTrafficLight(currentEgoPose, tlStopLinePosition, prevDistance, minTLDist)

%distanceToTrafficLight Compute distance to upcoming traffic light.

distance = ...
    helperSLComputeDistanceToTrafficLight(tlStopLinePosition, ...
    currentEgoPose, prevDistance, minTLDist);

== matlab function TLNWithUnrealTestBench/Sensors and Environment/StatetoNumber ==
  data: Labels input; D input; state output; distance_to_stop_line input
function state = StatetoNumber(Labels, D, distance_to_stop_line)
    % StatetoNumber converts the string to a number for the model to use

    % Initialize state to -1 (no detection) by default
    state = -1;
    fprintf('Calculated distance to the stop line: %.2f meters\n', D);
    %fprintf('Real distance to the stop line: %.2f meters\n', distance_to_stop_line);


    % Loop through the Labels
    for i = 1:length(Labels)
        if string(Labels(i)) == "Green_label"
            state = 2; % Green detected
        elseif string(Labels(i)) == "Yellow_label"
            state = 1; % Yellow detected
        elseif string(Labels(i)) == "Red_label"
            state = 0; % Red detected
    %Stop street if the scenario is load shedding
    %The model treats the no state condition as a red light when the
    %vehicle is 11 meters away. The vehicle then passes through the
    %intersection after stoping at the light
        elseif string(Labels(i)) == "NoState_label"
            if D <= 11;
                state = 0; % creating logic for red light braking
            end
        % elseif distance_to_stop_line == 0
        %     state = 2; %vehicle must go once stopped at traffic light 
        end 
        % If there is a detection, the state will be updated; otherwise, it remains -1.
        %display(Labels(i))
    end

== stateflow chart TLNWithUnrealTestBench/Sensors and Environment/Traffic Light Switching Logic ==
  state ENTER
    entry:
  state GREEN_STATE
    entry:
    tlState = Green;
  state YELLOW_STATE
    entry:
    tlState = Yellow;
  state RED_STATE
    entry:
    tlState = Red;
  (default) -> ENTER
  ENTER -> (junction 126) [order 2]
  (junction 126) -> RED_STATE : [[tlConfig.initialState == Red]]
  ENTER -> GREEN_STATE [order 1] : [[tlConfig.initialState == Green]]
  RED_STATE -> GREEN_STATE : after(5,sec)
  (junction 114) -> RED_STATE
  (junction 124) -> YELLOW_STATE
  YELLOW_STATE -> (junction 116)
  GREEN_STATE -> (junction 122) : after(5,sec)
  (junction 122) -> (junction 124) : [distanceToTL ~=0]
  (junction 116) -> (junction 114) : after(2,sec)
  data: tlState output =  tlConfig.initialState; Green constant double =2; Red constant double =0; Yellow constant double =1; distanceToTL input; tlConfig parameter

== matlab function TLNWithUnrealTestBench/Sensors and Environment/Traffic Light Select1 ==
  data: trafficLightId input; Labels input; state output
function state   = trafficLightSelect(trafficLightId, Labels)
%trafficLightSelect selects the traffic light that is under the control of
%ego vehicle and outputs its state.

% There are 30 traffic lights in US City Block scene. The valid
% traffic light ID will be in between 1 and 30.
if(trafficLightId >=1 && trafficLightId <= 30)
    % Get the upcomingTrafficLight state from the ground truth information
   % state = groundTruth(trafficLightId, 2);
   for i=1:length(Labels)
       state = Labels(i);
   end
else
    % If the upcomingTrafficLightId is 0 then the traffic light state is
    % set to -1 which is treated as no detection.
    state = -1;
end

end

== matlab function TLNWithUnrealTestBench/Sensors and Environment/Traffic Light Select2 ==
  data: trafficLightId input; state input; state output
function state   = trafficLightSelect(trafficLightId, state)
%trafficLightSelect selects the traffic light that is under the control of
%ego vehicle and outputs its state.

% There are 30 traffic lights in US City Block scene. The valid
% traffic light ID will be in between 1 and 30.
if(trafficLightId >=1 && trafficLightId <= 30)
    % Get the upcomingTrafficLight state from the ground truth information
    state = state;
    display(state)
else
    % If the upcomingTrafficLightId is 0 then the traffic light state is
    % set to -1 which is treated as no detection.
    state = -1;
end

end
